simulink model "mavsim_chap5"  (R2018b)
settings: Solver=ode45  StartTime=0.0  StopTime=10000  RelTol=1e-3  EnableMultiTasking=on
InitFcn:
  | param_chap5
  | aerosonde
undefined symbols (not defined in the file or in its folder): drawVehicle, forces_moments, HDBK, Light, MIL, Newton, P, plotmavstatevariables, Raphson, u_trim
libraries: aerolibwind2 x2, aerolibobsolete x1
settings Model: Creator=beard  LastModifiedBy=xinyizhao
settings DataIOCC: LimitDataPoints=on  SaveFormat=Array  SignalLoggingSaveFormat=ModelDataLogs
settings OptimizationCC: ExpressionDepthLimit=2147483647  InitFltsAndDblsToZero=on  LifeSpan=inf
settings DebuggingCC: UnderspecifiedInitializationDetection=Classic  MergeDetectMultiDrivingBlocksExec=none  SolverPrmCheckMsg=warning  FcnCallInpInsideContextMsg=warning  StateNameClashWarn=warning  LibraryContextMissingDiagnostic=none  SFUnexpectedBacktrackingDiag=warning  SFNoUnconditionalDefaultTransitionDiag=warning  SFExecutionAtInitializationDiag=none
settings HardwareCC: ProdBitPerPointer=32  ProdBitPerSizeT=32  ProdBitPerPtrDiffT=32  ProdLargestAtomicFloat=None  ProdIntDivRoundTo=Undefined  ProdEndianess=Unspecified  ProdWordSize=32  ProdHWDeviceType=32-bit Generic
settings ModelReferenceCC: PropagateSignalLabelsOutOfModel=off
settings SFSimCC: SimUseLocalCustomCode=off
settings RTWCC: RTWUseLocalCustomCode=off
settings CodeAppCC: StateflowObjectComments=on
settings GRTTargetCC: TargetLangStandard=C89/C90 (ANSI)  GeneratePreprocessorConditionals=Disable all  CombineOutputUpdateFcns=off  GRTInterface=on
settings ConfigComp: CovMetricSettings=dw  CovHtmlReporting=on  CovSaveCumulativeToWorkspaceVar=on  CovSaveSingleToWorkspaceVar=on  CovExternalEMLEnable=off  CovSFcnEnable=off

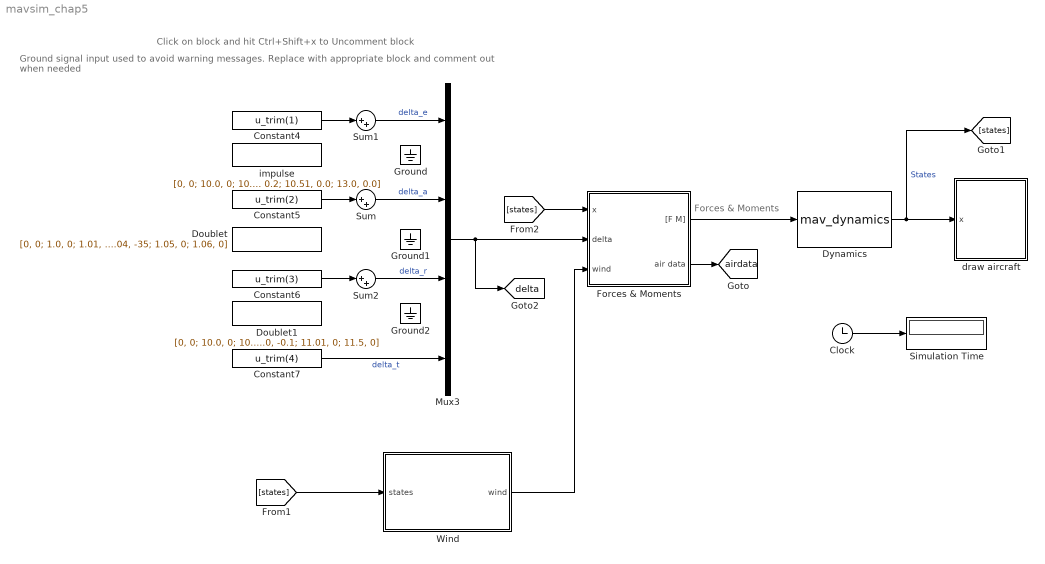
== system mavsim_chap5 ==
  note: Ground signal input used to avoid warning messages. Replace with appropriate block and comment out when needed
  note: Click on block and hit Ctrl+Shift+x to Uncomment block
  note: Forces & Moments
  Clock : Clock
  Constant4 : Constant  Value=u_trim(1)
  Constant5 : Constant  Value=u_trim(2)
  Constant6 : Constant  Value=u_trim(3)
  Constant7 : Constant  Value=u_trim(4)
  Doublet : FromWorkspace  VariableName=[0, 0; 1.0, 0; 1.01, 35; 1.02, 35; 1.03, -35; 1.04, -35; 1.05, 0; 1.06, 0]  SampleTime=0
  Doublet1 : FromWorkspace  VariableName=[0, 0; 10.0, 0; 10.01, 0.1; 10.5, 0.1; 10.51, -0.1; 11.0, -0.1; 11.01, 0; 11.5, 0]  SampleTime=0
  Dynamics : S-Function  FunctionName=mav_dynamics  Parameters=P  SFunctionDeploymentMode=off  EnableBusSupport=off
  Forces & Moments : Subsystem
  Ground : Ground
  Ground1 : Ground
  Ground2 : Ground
  Mux3 : Mux
  Simulation Time : Display
  Sum : Sum  Inputs=|++
  Sum1 : Sum  Inputs=|++
  Sum2 : Sum  Inputs=|++
  Wind : Subsystem
  draw aircraft : Subsystem
      mask Display: image(imread('tv.jpg'))
  impulse : FromWorkspace  VariableName=[0, 0; 10.0, 0; 10.01, 0.2; 10.5, 0.2; 10.51, 0.0; 13.0, 0.0]  SampleTime=0
  tag scope: airdata=global, delta=global
  wires:
  Dynamics/1 -> draw aircraft/1(x), [states]  "States"
  Forces & Moments/1("[F M]") -> Dynamics/1
  Clock/1 -> Simulation Time/1
  Forces & Moments/2(air data) -> [airdata]
  Constant5/1 -> Sum/1
  Constant4/1 -> Sum1/1
  Constant6/1 -> Sum2/1
  Sum1/1 -> Mux3/1  "delta_e"
  Sum/1 -> Mux3/2  "delta_a"
  Sum2/1 -> Mux3/3  "delta_r"
  Constant7/1 -> Mux3/4  "delta_t"
  Wind/1(wind) -> Forces & Moments/3(wind)
  [states] -> Wind/1(states)
  Mux3/1 -> [delta], Forces & Moments/2(delta)
  [states] -> Forces & Moments/1(x)

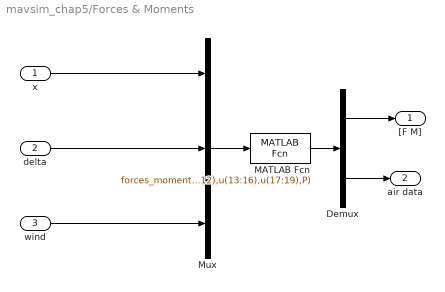
== system mavsim_chap5/Forces & Moments ==
  x : Inport
  delta : Inport  Port=2
  wind : Inport  Port=3
  Demux : Demux  Outputs=[6;6]
  MATLAB Fcn : MATLABFcn  MATLABFcn=forces_moments(u(1:12),u(13:16),u(17:19),P)  OutputDimensions=12
  Mux : Mux  Inputs=3
  "[F M]" : Outport
  air data : Outport  Port=2
  wires:
  x/1 -> Mux/1
  delta/1 -> Mux/2
  wind/1 -> Mux/3
  MATLAB Fcn/1 -> Demux/1
  Demux/1 -> "[F M]"/1
  Mux/1 -> MATLAB Fcn/1
  Demux/2 -> air data/1

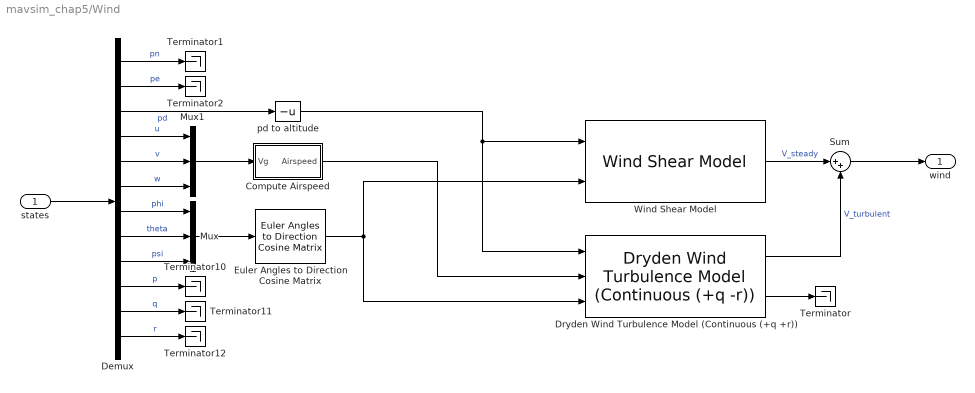
== system mavsim_chap5/Wind ==
  states : Inport
  Compute Airspeed : Subsystem
  Demux : Demux  Outputs=12
  Dryden Wind Turbulence Model (Continuous (+q +r)) : aerolibwind2/Dryden Wind Turbulence Model  (Continuous (+q -r))  units=Metric (MKS)  spec=MIL-HDBK-1797  model=Continuous Dryden (+q +r)  W20=P.w_mag  Wdeg=P.w_dir  TurbProb=10^-2 - Light  L_high=533.4  Wingspan=P.b  ts=0.1  Seed=[23341 23342 0 23344]  T_on=off
      settings: SourceProductName=Aerospace Blockset
  Euler Angles to Direction Cosine Matrix : aerolibobsolete/Euler Angles to  Direction Cosine Matrix
      settings: SourceProductName=Aerospace Blockset  SourceProductBaseCode=AE
  Mux : Mux  Inputs=3
  Mux1 : Mux  Inputs=3
  Sum : Sum  Inputs=|++
  Terminator{,1..2,10..12} (6 alike) : Terminator
  Wind Shear Model : aerolibwind2/Wind Shear Model  units=Metric (MKS)  phase=Category C - Terminal Flight Phase  W_20=P.w_mag  Wdeg=P.w_dir
      settings: SourceProductName=Aerospace Blockset
  pd to altitude : UnaryMinus
  wind : Outport
  wires:
  Dryden Wind Turbulence Model (Continuous (+q +r))/2 -> Terminator/1
  Euler Angles to Direction Cosine Matrix/1 -> Dryden Wind Turbulence Model (Continuous (+q +r))/3, Wind Shear Model/2
  Wind Shear Model/1 -> Sum/1  "V_steady"
  Compute Airspeed/1(Airspeed) -> Dryden Wind Turbulence Model (Continuous (+q +r))/2
  pd to altitude/1 -> Wind Shear Model/1, Dryden Wind Turbulence Model (Continuous (+q +r))/1
  Dryden Wind Turbulence Model (Continuous (+q +r))/1 -> Sum/2  "V_turbulent"
  states/1 -> Demux/1
  Demux/1 -> Terminator1/1  "pn"
  Demux/2 -> Terminator2/1  "pe"
  Demux/3 -> pd to altitude/1  "pd"
  Demux/4 -> Mux1/1  "u"
  Demux/5 -> Mux1/2  "v"
  Demux/6 -> Mux1/3  "w"
  Demux/7 -> Mux/1  "phi"
  Demux/8 -> Mux/2  "theta"
  Demux/9 -> Mux/3  "psi"
  Demux/10 -> Terminator10/1  "p"
  Demux/11 -> Terminator11/1  "q"
  Demux/12 -> Terminator12/1  "r"
  Mux/1 -> Euler Angles to Direction Cosine Matrix/1
  Mux1/1 -> Compute Airspeed/1(Vg)
  Sum/1 -> wind/1

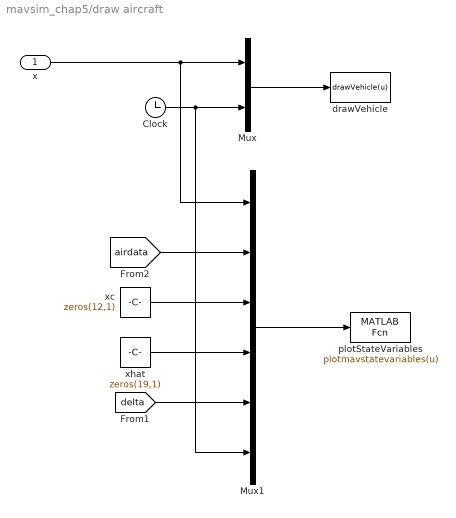
== system mavsim_chap5/draw aircraft ==
  x : Inport
  Clock : Clock
  Mux : Mux  Inputs=2
  Mux1 : Mux  Inputs=6
  drawVehicle : MATLABFcn  MATLABFcn=drawVehicle(u)  OutputDimensions=0  SampleTime=0.1
  plotStateVariables : MATLABFcn  MATLABFcn=plotmavstatevariables(u)  OutputDimensions=0  SampleTime=0.1
  xc : Constant  Value=zeros(12,1)
  xhat : Constant  Value=zeros(19,1)
  wires:
  [airdata] -> Mux1/2
  [delta] -> Mux1/5
  xc/1 -> Mux1/3
  xhat/1 -> Mux1/4
  Mux1/1 -> plotStateVariables/1
  Clock/1 -> Mux1/6, Mux/2
  x/1 -> Mux1/1, Mux/1
  Mux/1 -> drawVehicle/1

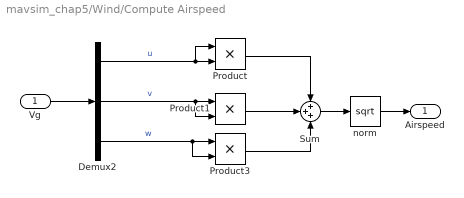
== system mavsim_chap5/Wind/Compute Airspeed ==
  Vg : Inport
  Demux2 : Demux  Outputs=3
  Product : Product  RndMeth=Zero
  Product1 : Product  RndMeth=Zero
  Product3 : Product  RndMeth=Zero
  Sum : Sum  Inputs=+++
  norm : Sqrt  AlgorithmType=Newton-Raphson  SaturateOnIntegerOverflow=on
  Airspeed : Outport
  wires:
  Vg/1 -> Demux2/1
  Product/1 -> Sum/1
  Sum/1 -> norm/1
  Demux2/1 -> Product/2, Product/1  "u"
  Product1/1 -> Sum/2
  Product3/1 -> Sum/3
  Demux2/2 -> Product1/2, Product1/1  "v"
  Demux2/3 -> Product3/2, Product3/1  "w"
  norm/1 -> Airspeed/1
